simulink model "manual_PID"  (R2019b)
settings: Solver=VariableStepAuto  StartTime=0.0  StopTime=10.0  RelTol=1e-3
undefined symbols (not defined in the file or in its folder): cz_ratio, dt_control, PARAMS, pc_ratio, wc
settings Model: Creator=francescoceresetti  LastModifiedBy=francescoceresetti

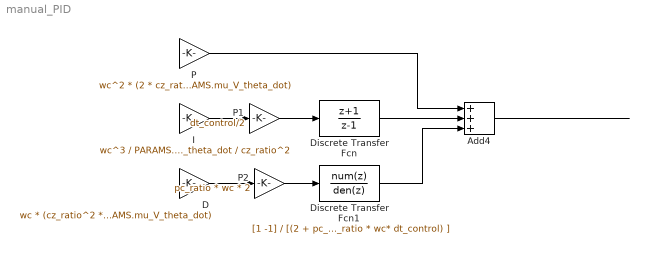
== system manual_PID ==
  Add4 : Sum  Inputs=+++
  D : Gain  Gain="wc * (cz_ratio^2 * pc_ratio^2 - 2 * cz_ratio * pc_ratio + 1)  / (cz_ratio^2 * pc_ratio^2 * PARAMS.mu_V_theta_dot)"
  Discrete Transfer Fcn : DiscreteTransferFcn  Numerator=[1 1]  Denominator=[1 -1]
  Discrete Transfer Fcn1 : DiscreteTransferFcn  Numerator=[1 -1]  Denominator=[(2 + pc_ratio * wc * dt_control) (-2 + pc_ratio * wc* dt_control) ]
  I : Gain  Gain=wc^3 / PARAMS.mu_V_theta_dot / cz_ratio^2
  P : Gain  Gain=wc^2 * (2 * cz_ratio * pc_ratio - 1) / (cz_ratio^2 * pc_ratio * PARAMS.mu_V_theta_dot)
  P1 : Gain  Gain=dt_control/2
  P2 : Gain  Gain=pc_ratio * wc * 2
  wires:
  P2/1 -> Discrete Transfer Fcn1/1
  Discrete Transfer Fcn/1 -> Add4/2
  P/1 -> Add4/1
  ? -> D/1, P/1, I/1
  D/1 -> P2/1
  Discrete Transfer Fcn1/1 -> Add4/3
  P1/1 -> Discrete Transfer Fcn/1
  I/1 -> P1/1
  Add4/1 -> ?
